simulink model "main_sim"  (R2022b)
settings: Solver=VariableStepAuto  StartTime=0.0  StopTime=stop_time  FixedStep=0.1  RelTol=1e-3
values from neighbouring files (symbols this model uses):
  M = 8    [params.m]
  SA_minimum_samples = 2^10    (= 1024)    [params.m]
  sample_time = 1/fs    (= 8.14332247557e-09)    [params.m]
undefined symbols (not defined in the file or in its folder): magnitude, QAM
libraries: whdlmod x2, simulink x1, commrandsrc3 x1
settings Model: Creator=mchubashi  LastModifiedBy=mchubashi

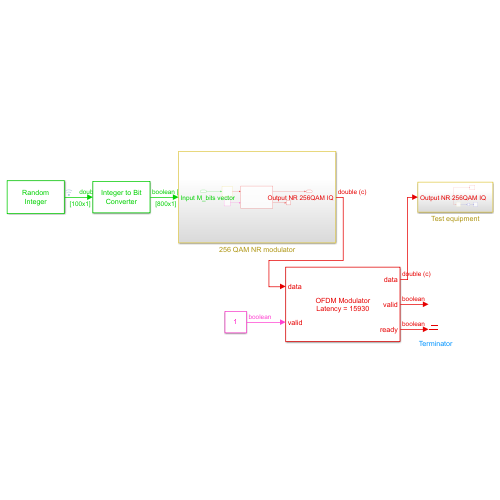
[thumbnail: Simulink's stored preview of the top-level diagram]
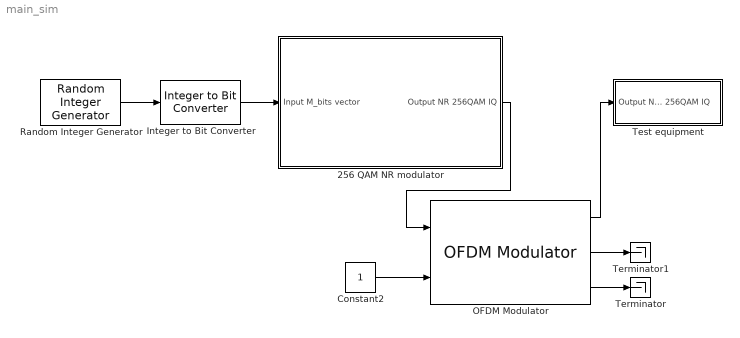
== system main_sim ==
  256 QAM NR modulator : Subsystem
  Constant2 : Constant  OutDataTypeStr=boolean
  Integer to Bit Converter : simulink/Logic and Bit Operations/Integer to Bit Converter  nbits=M  signedInputValues=Unsigned  bitOrder=MSB first  outDtype=boolean
  OFDM Modulator : whdlmod/OFDM Modulator  OFDMParametersSource=Property  FFTLength=OFDM_FFT_size  MaxFFTLength=64  CPLength=cp_samples  numLgSc=half_guard_samples  numRgSc=half_guard_samples  InsertDCNull=off  Windowing=on  WindowLength=4  MaxWindowLength=8  ResetInputPort=off  Normalize=on  RoundingMethod=Floor  SimulateUsing=Code generation
  Random Integer Generator : commrandsrc3/Random Integer Generator  SetSize=2^M  SeedSource=Auto  Seed=0  SampleTime=sample_time  SamplesPerFrame=samples_per_frame  OutputDataType=double  SimulateUsing=Interpreted execution
  Terminator : Terminator
  Terminator1 : Terminator
  Test equipment : Subsystem
  wires:
  Random Integer Generator/1 -> Integer to Bit Converter/1
  Integer to Bit Converter/1 -> 256 QAM NR modulator/1(Input M_bits vector)
  256 QAM NR modulator/1(Output NR 256QAM IQ) -> OFDM Modulator/1
  OFDM Modulator/3 -> Terminator/1
  OFDM Modulator/2 -> Terminator1/1
  Constant2/1 -> OFDM Modulator/2
  OFDM Modulator/1 -> Test equipment/1(Output NR 256QAM IQ)

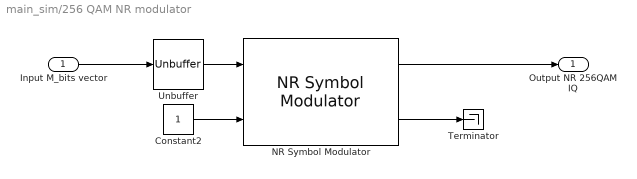
== system main_sim/256 QAM NR modulator ==
  Input M_bits vector : Inport
  Constant2 : Constant  OutDataTypeStr=boolean
  NR Symbol Modulator : whdlmod/NR Symbol Modulator  ModulationSource=Property  ModulationScheme=256-QAM  SimulateUsing=Code generation  OutputDataType=double  WordLength=16
  Terminator : Terminator
  Unbuffer : Unbuffer
  Output NR 256QAM IQ : Outport
  wires:
  Constant2/1 -> NR Symbol Modulator/2
  Unbuffer/1 -> NR Symbol Modulator/1
  NR Symbol Modulator/1 -> Output NR 256QAM IQ/1
  NR Symbol Modulator/2 -> Terminator/1
  Input M_bits vector/1 -> Unbuffer/1

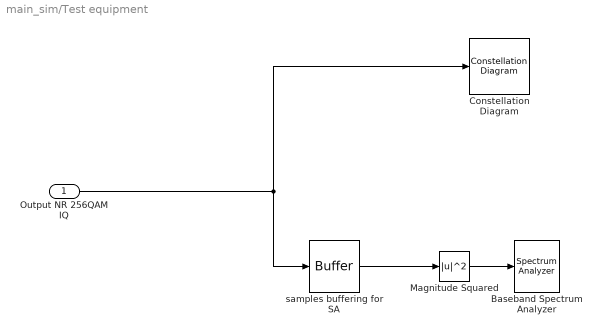
== system main_sim/Test equipment ==
  Output NR 256QAM IQ : Inport
  Baseband Spectrum Analyzer : SpectrumAnalyzer
  Constellation Diagram : ConstellationDiagram  WindowPosition=[1080.000000,165.000000,600.000000,600.000000,]  ScopeFrameLocation=window  ReferenceConstellation=256-QAM  DefaultConfigurationName=comm.scopes.ConstellationDiagramBlockCfg
  Magnitude Squared : Math  Operator=magnitude^2
  samples buffering for SA : Buffer  N=SA_minimum_samples  OutputFrames=off
  wires:
  samples buffering for SA/1 -> Magnitude Squared/1
  Magnitude Squared/1 -> Baseband Spectrum Analyzer/1
  Output NR 256QAM IQ/1 -> samples buffering for SA/1, Constellation Diagram/1
